simulink model "Ass2_Ex2_Part2_sim"  (R2024a)
settings: Solver=ode15s  StartTime=0  StopTime=16239.0058  MaxStep=1e-2  RelTol=1e-10  AbsTol=1e-12
values from neighbouring files (symbols this model uses):
  K = constant()    [Pareschi252142_Assign2_Ex1.m]    (also in Pareschi252142_Assign2_Ex2.m)
  x0 = [298.15 * ones(5, 1); -0.4 * pi; 0; 0]    [Pareschi252142_Assign2_Ex1.m]    (also in Pareschi252142_Assign2_Ex2.m = [0; 0; 0.75*K.xv_max; 0; 0])
libraries: fl_lib x29, nesl_utility x8, ee_lib x1
settings Model: Creator=marcellopareschi  LastModifiedBy=marcellopareschi
settings SolverCC: AutoScaleAbsTol=off  AlgebraicLoopSolver=TrustRegion  MaxZcPerStep=1
settings DebuggingCC: UnconnectedInputMsg=warning  UnconnectedOutputMsg=warning  UnconnectedLineMsg=warning  SymbolicDimsDataTypeCodeGenerationDiagnostic=none
settings ModelReferenceCC: EnableRefExpFcnMdlSchedulingChecks=on
settings SFSimCC: CustomCodeUndefinedFunction=UseInterfaceOnly
settings RTWCC: GPUComputeCapability=3.5  DLArmComputeVersion=19.05
settings SimscapeCC: SimscapeLogType=all  SimscapeLogSimulationStatistics=on  SimscapeLogDataHistory=10000

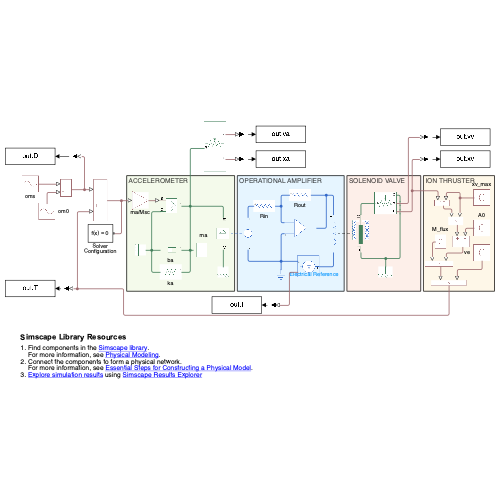
[thumbnail: Simulink's stored preview of the top-level diagram]
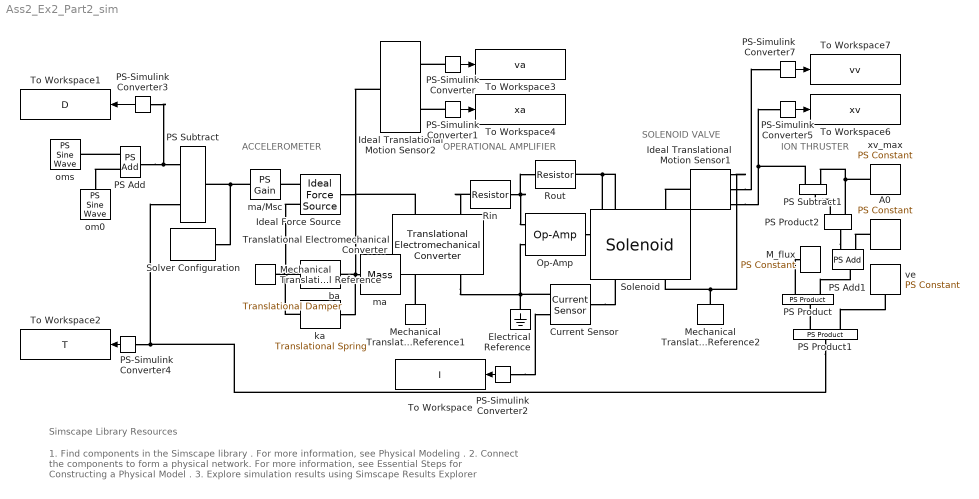
== system Ass2_Ex2_Part2_sim ==
  note: ION THRUSTER
  note: SOLENOID VALVE
  note: OPERATIONAL AMPLIFIER
  note: ACCELEROMETER
  note: 1. Find components in the Simscape library .
      | For more information, see Physical Modeling .
      | 2. Connect the components to form a physical network.
      | For more information, see Essential Steps for Constructing a Physical Model .
      | 3. Explore simulation results using Simscape Results Explorer
  note: Simscape Library Resources
  A0 : fl_lib/Physical Signals/Sources/PS Constant  constant=K.A0 m^2
  Current Sensor : fl_lib/Electrical/Electrical Sensors/Current Sensor
  Electrical Reference : fl_lib/Electrical/Electrical Elements/Electrical Reference
  Ideal Force Source : fl_lib/Mechanical/Mechanical Sources/Ideal Force Source
  Ideal Translational Motion Sensor1 : fl_lib/Mechanical/Mechanical Sensors/Ideal Translational Motion Sensor  reference=foundation.enum.MeasurementReference.difference  acceleration_port=false  velocity_port=true  position_port=true  offset=0 m
  Ideal Translational Motion Sensor2 : fl_lib/Mechanical/Mechanical Sensors/Ideal Translational Motion Sensor  reference=foundation.enum.MeasurementReference.absolute  acceleration_port=false  velocity_port=true  position_port=true  offset=0 m
      settings: InternalSimscapePortConfiguration="{\"Bottom\":[],\"Left\":[{\"id\":\"R\",\"label\":\"R\",\"type\":\"foundation.mechanical.translational.translational\"}],\"Right\":[{\"id\":\"V\",\"label\":\"V\",\"type\":\"output\"},{\"id\":\"P\",\"label\":\"P\",\"type\":\"output\"}],\"Top\":[]}"
  M_flux : fl_lib/Physical Signals/Sources/PS Constant  constant=K.M_flux N*s/m^3
  Mechanical Translational Reference : fl_lib/Mechanical/Translational Elements/Mechanical Translational Reference
  Mechanical Translational Reference1 : fl_lib/Mechanical/Translational Elements/Mechanical Translational Reference
  Mechanical Translational Reference2 : fl_lib/Mechanical/Translational Elements/Mechanical Translational Reference
  Op-Amp : fl_lib/Electrical/Electrical Elements/Op-Amp  outI_specify=off  outI_priority=None  outI=0 A  outI_nominal_specify=off  outI_nominal_value=1  outI_nominal_unit=A
  PS Add : fl_lib/Physical Signals/Functions/PS Add
  PS Add1 : fl_lib/Physical Signals/Functions/PS Add
  PS Product : fl_lib/Physical Signals/Functions/PS Product
  PS Product1 : fl_lib/Physical Signals/Functions/PS Product
  PS Product2 : fl_lib/Physical Signals/Functions/PS Product
  PS Subtract : fl_lib/Physical Signals/Functions/PS Subtract
  PS Subtract1 : fl_lib/Physical Signals/Functions/PS Subtract
  PS-Simulink Converter{,1..5,7} (7 alike) : nesl_utility/PS-Simulink Converter  PhysicalDomain=network_engine_domain  SubClassName=ps_output  LeftPortType=input  RightPortType=output  PseudoPeriodic=off  Frequencies=[]  VectorFormat=inherit  Unit=inherit  AffineConversion=off
  Rin : fl_lib/Electrical/Electrical Elements/Resistor  R=K.Rin_min Ohm  i_specify=off  i_priority=None  i=0 A  i_nominal_specify=off  i_nominal_value=1  i_nominal_unit=A  v_specify=off  v_priority=None  v=0 V  v_nominal_specify=off  v_nominal_value=1  v_nominal_unit=V
  Rout : fl_lib/Electrical/Electrical Elements/Resistor  R=K.Rf_max Ohm  i_specify=off  i_priority=None  i=0 A  i_nominal_specify=off  i_nominal_value=1  i_nominal_unit=A  v_specify=off  v_priority=None  v=0 V  v_nominal_specify=off  v_nominal_value=1  v_nominal_unit=V
  Solenoid : ee_lib/Electromechanical/Mechatronic Actuators/Solenoid  motionDirection=ee.enum.actuators.solenoidDirection.away  F12=[9000, 12] N  X12=[0, 0.1] mm  Vdc=0.6 mV  Imax=0.1 A  K=K.kv N/m  Xzero=0 mm  lam=K.bv N*s/m  Mass=K.mv kg  Xmax=0.1 mm  K_endstop=0.12*1e6 N/m  D_endstop=1e4 N*s/m  i_specify=on  i_priority=High  i=0 A  i_nominal_specify=off  i_nominal_value=1  i_nominal_unit=A  x_specify=on  x_priority=High  x=K.xv_max*0.75 m  x_nominal_specify=off  x_nominal_value=1  x_nominal_unit=mm  vel_specify=on  vel_priority=High  vel=0 m/s  vel_nominal_specify=off  vel_nominal_value=1  vel_nominal_unit=mm/s  F_specify=off  F_priority=None  F=0 N  F_nominal_specify=off  F_nominal_value=1  F_nominal_unit=N  v_L_specify=off  v_L_priority=None  v_L=0 V  v_L_nominal_specify=off  v_L_nominal_value=1  v_L_nominal_unit=V  magnetic_force_specify=off  magnetic_force_priority=None  magnetic_force=0 N  magnetic_force_nominal_specify=off  magnetic_force_nominal_value=1  magnetic_force_nominal_unit=N  alpha=3.93e-3 1/K  Tmeas=25 degC  thermal_mass=100 J/K  temperature_specify=off  temperature_priority=High  temperature=25 degC  temperature_nominal_specify=off  temperature_nominal_value=1  temperature_nominal_unit=degC  Q_specify=off  Q_priority=None  Q=0 W  Q_nominal_specify=off  Q_nominal_value=1  Q_nominal_unit=W
      settings: InternalSimscapePortConfiguration="{\"Bottom\":[],\"Left\":[{\"id\":\"p\",\"label\":\"+\",\"type\":\"foundation.electrical.electrical\"},{\"id\":\"R\",\"label\":\"R\",\"type\":\"foundation.mechanical.translational.translational\"}],\"Right\":[{\"id\":\"n\",\"label\":\"-\",\"type\":\"foundation.electrical.electrical\"},{\"id\":\"C\",\"label\":\"C\",\"type\":\"foundation.mechanical.translational.translational\"}],\"Top\":[]}"
  Solver Configuration : nesl_utility/Solver Configuration  PhysicalDomain=network_engine_domain  SubClassName=solver  LeftPortType=input  RightPortType=generic  Tones=[]  Harmonics=[]  SimulateNoise=off  Profile=off  UseLocalSampling=off  EnableSwitchedLinearOptims=on  FrequencyDomain=off  UseCCode=off  RelTol=0.001  AbsTol=1e-06  MinStep=1e-09  ToWorkspace=off  RevertToSquareIcSolve=off  NumHomotopyIterations=100  PhasorMode=off  PhasorModeNumHarmonics=1  ConsistencySolver=NEWTON_XTOL_AFTER_FTOL  IndexReductionMethod=DerivativeReplacement  DoDC=off  ResidualTolerance=1e-09  ConsistencyTolSource=GLOBAL  ConsistencyAbsTol=0.001  ConsistencyRelTol=0.001  ConsistencyTolFactor=0.001  UseLocalSolver=off  LocalSolverChoice=NE_BACKWARD_EULER_ADVANCER  ResolveIndetEquations=on  FunctionEvalNumThread=1  LocalSolverSampleTime=0.001  DoFixedCost=off  MaxNonlinIter=3  MaxModeIter=2  ComputeImpulses=off  ImpulseIterations=2  LinearAlgebra=auto  LinearAlgebraNumThread=0  EquationFormulation=NE_TIME_EF  DelaysMemoryBudget=1024  AutomaticFiltering=on  FilteringTimeConstant=0.001  PartitionStorageMethod=AS_NEEDED  PartitionMemoryBudget=1024  PartitionMethod=ROBUST  MultibodyUseLocalSolver=off  MultibodyLocalSolverChoice=ODE1  MultibodyLocalSolverSampleTime=0.001
  To Workspace : ToWorkspace  VariableName=I  SampleTime=-1
  To Workspace1 : ToWorkspace  VariableName=D  SampleTime=-1
  To Workspace2 : ToWorkspace  VariableName=T  SampleTime=-1
  To Workspace3 : ToWorkspace  VariableName=va  SampleTime=-1
  To Workspace4 : ToWorkspace  VariableName=xa  SampleTime=-1
  To Workspace6 : ToWorkspace  VariableName=xv  SampleTime=-1
  To Workspace7 : ToWorkspace  VariableName=vv  SampleTime=-1
  Translational Electromechanical Converter : fl_lib/Electrical/Electrical Elements/Translational Electromechanical Converter  K=K.Kacc V*s/m  i_specify=off  i_priority=None  i=0 A  i_nominal_specify=off  i_nominal_value=1  i_nominal_unit=A  v_specify=off  v_priority=None  v=0 V  v_nominal_specify=off  v_nominal_value=1  v_nominal_unit=V  f_specify=off  f_priority=None  f=0 N  f_nominal_specify=off  f_nominal_value=1  f_nominal_unit=N  u_specify=off  u_priority=None  u=0 m/s  u_nominal_specify=off  u_nominal_value=1  u_nominal_unit=m/s
      settings: InternalSimscapePortConfiguration="{\"Bottom\":[],\"Left\":[{\"id\":\"p\",\"label\":\"+\",\"type\":\"foundation.electrical.electrical\"},{\"id\":\"R\",\"label\":\"R\",\"type\":\"foundation.mechanical.translational.translational\"}],\"Right\":[{\"id\":\"n\",\"label\":\"-\",\"type\":\"foundation.electrical.electrical\"},{\"id\":\"C\",\"label\":\"C\",\"type\":\"foundation.mechanical.translational.translational\"}],\"Top\":[]}"
  ba : fl_lib/Mechanical/Translational Elements/Translational Damper  D=K.ba_min N*s/m  v_specify=off  v_priority=None  v=x0(2) m/s  v_nominal_specify=off  v_nominal_value=1  v_nominal_unit=m/s  f_specify=off  f_priority=None  f=0 N  f_nominal_specify=off  f_nominal_value=1  f_nominal_unit=N
  ka : fl_lib/Mechanical/Translational Elements/Translational Spring  spr_rate=K.ka_max N/m  v_specify=on  v_priority=High  v=0 m/s  v_nominal_specify=off  v_nominal_value=1  v_nominal_unit=m/s  f_specify=off  f_priority=None  f=0 N  f_nominal_specify=off  f_nominal_value=1  f_nominal_unit=N  x_specify=on  x_priority=High  x=0 m  x_nominal_specify=off  x_nominal_value=1  x_nominal_unit=m
  ma : fl_lib/Mechanical/Translational Elements/Mass  mass=K.ma kg  num_ports=foundation.enum.numPorts2.one  v_specify=off  v_priority=High  v=0 m/s  v_nominal_specify=off  v_nominal_value=1  v_nominal_unit=m/s  f_specify=off  f_priority=None  f=0 N  f_nominal_specify=off  f_nominal_value=1  f_nominal_unit=N
  ma/Msc : fl_lib/Physical Signals/Functions/PS Gain  gain=K.ma/K.Msc
  om0 : fl_lib/Physical Signals/Sources/PS Sine Wave  amplitude=0.6 mN  bias=0  frequency_spec=foundation.enum.frequencySpec.angular  frequency_SI=2*K.om0 Hz  frequency_angular=2*K.om0 rad/s  phase=0 rad
      settings: InternalSimscapePortConfiguration="{\"Bottom\":[],\"Left\":[],\"Right\":[{\"id\":\"O\",\"label\":\"\",\"type\":\"output\"}],\"Top\":[]}"
  oms : fl_lib/Physical Signals/Sources/PS Sine Wave  amplitude=1 mN  bias=2.2 mN  frequency_spec=foundation.enum.frequencySpec.angular  frequency_SI=K.oms GHz  frequency_angular=K.oms rad/s  phase=-pi/2 rad
      settings: InternalSimscapePortConfiguration="{\"Bottom\":[],\"Left\":[],\"Right\":[{\"id\":\"O\",\"label\":\"\",\"type\":\"output\"}],\"Top\":[]}"
  ve : fl_lib/Physical Signals/Sources/PS Constant  constant=K.ve m/s
  xv_max : fl_lib/Physical Signals/Sources/PS Constant  constant=K.xv_max m
  wires:
  PS-Simulink Converter7/1 -> To Workspace7/1
  PS-Simulink Converter5/1 -> To Workspace6/1
  PS-Simulink Converter/1 -> To Workspace3/1
  PS-Simulink Converter1/1 -> To Workspace4/1
  PS-Simulink Converter2/1 -> To Workspace/1
  PS-Simulink Converter3/1 -> To Workspace1/1
  PS-Simulink Converter4/1 -> To Workspace2/1
  connections:
  Rin/LConn1 -- Translational Electromechanical Converter/LConn1
  ba/RConn1 -- Mechanical Translational Reference/LConn1 -- Ideal Force Source/RConn2 -- ka/RConn1
  ka/LConn1 -- ma/LConn1 -- Ideal Translational Motion Sensor2/LConn1 -- Translational Electromechanical Converter/LConn2 -- Ideal Force Source/LConn1 -- ba/LConn1
  Mechanical Translational Reference1/LConn1 -- Translational Electromechanical Converter/RConn2
  Ideal Force Source/RConn1 -- ma/Msc/RConn1
  Solenoid/LConn1 -- Op-Amp/RConn1 -- Rout/RConn1
  Rin/RConn1 -- Rout/LConn1 -- Op-Amp/LConn2
  Mechanical Translational Reference2/LConn1 -- Ideal Translational Motion Sensor1/RConn1 -- Solenoid/RConn2
  Ideal Translational Motion Sensor1/LConn1 -- Solenoid/LConn2
  Ideal Translational Motion Sensor1/RConn2 -- PS-Simulink Converter7/LConn1
  ma/Msc/LConn1 -- PS Subtract/RConn1 -- Solver Configuration/RConn1
  Ideal Translational Motion Sensor1/RConn3 -- PS Subtract1/LConn2 -- PS-Simulink Converter5/LConn1
  PS Add/LConn2 -- om0/RConn1
  PS Add/LConn1 -- oms/RConn1
  PS Add/RConn1 -- PS Subtract/LConn2 -- PS-Simulink Converter3/LConn1
  PS-Simulink Converter/LConn1 -- Ideal Translational Motion Sensor2/RConn1
  PS-Simulink Converter1/LConn1 -- Ideal Translational Motion Sensor2/RConn2
  Translational Electromechanical Converter/RConn1 -- Electrical Reference/LConn1 -- Current Sensor/RConn2 -- Op-Amp/LConn1
  PS Product2/LConn1 -- PS Subtract1/RConn1
  PS Product1/LConn1 -- ve/RConn1
  PS Product1/LConn2 -- PS Product/RConn1
  PS Product/LConn1 -- PS Add1/RConn1
  PS Product/LConn2 -- M_flux/RConn1
  PS Product1/RConn1 -- PS-Simulink Converter4/LConn1 -- PS Subtract/LConn1
  PS-Simulink Converter2/LConn1 -- Current Sensor/RConn1
  xv_max/RConn1 -- PS Subtract1/LConn1 -- PS Product2/LConn2
  A0/RConn1 -- PS Add1/LConn1
  PS Product2/RConn1 -- PS Add1/LConn2
  Current Sensor/LConn1 -- Solenoid/RConn1
